simulink model "FOCControlDiscreteModel"  (R2022a)
settings: Solver=FixedStepDiscrete  StartTime=0.0  StopTime=2  RelTol=1e-3  EnableMultiTasking=on
values from neighbouring files (symbols this model uses):
  Ki_current = 6.0    (= 6)    [FOCControlDiscrete.m]
  Ki_speed = 6.0    (= 6)    [FOCControlDiscrete.m]
  Kp_current = 12.0    (= 12)    [FOCControlDiscrete.m]
  Kp_speed = 0.459    [FOCControlDiscrete.m]
  P = 6    [FOCControlDiscrete.m]
  Ts_current_control_loop = 30e-6    (= 3e-05)    [FOCControlDiscrete.m]
  Ts_speed_control_loop = 2 * Ts_observer    (= 0.00012)    [FOCControlDiscrete.m]
  Vdc = 12    [FOCControlDiscrete.m]
undefined symbols (not defined in the file or in its folder): Ts_motor
libraries: mcbcontrolslib x6, slpidlib x3, mcbpositiondecoderlib x3, simulink_extras x2, mcbplantlib x1, autolibpmsmexterior x1
settings Model: Creator=brandon  LastModifiedBy=brandon
settings SolverCC: AutoInsertRateTranBlk=on
settings DebuggingCC: ParameterPrecisionLossMsg=none

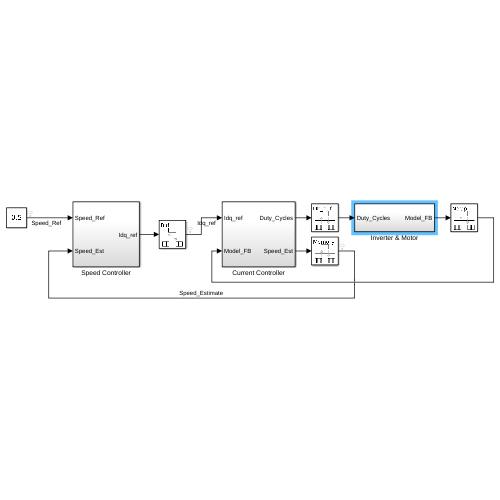
[thumbnail: Simulink's stored preview of the top-level diagram]
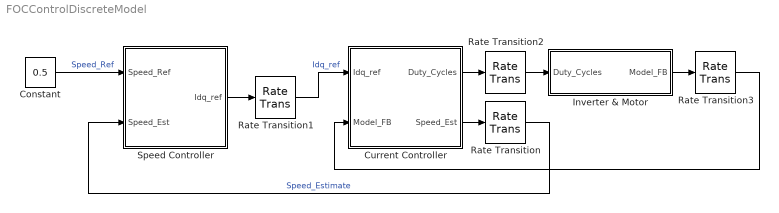
== system FOCControlDiscreteModel ==
  Constant : Constant  Value=0.5  OutDataTypeStr=single
  Current Controller : Subsystem
  Inverter & Motor : Subsystem
  Rate Transition{,1..3} (4 alike) : RateTransition  Deterministic=off
  Speed Controller : Subsystem
  wires:
  Constant/1 -> Speed Controller/1(Speed_Ref)  "Speed_Ref"
  Rate Transition/1 -> Speed Controller/2(Speed_Est)  "Speed_Estimate"
  Speed Controller/1(Idq_ref) -> Rate Transition1/1
  Rate Transition1/1 -> Current Controller/1(Idq_ref)  "Idq_ref"
  Current Controller/1(Duty_Cycles) -> Rate Transition2/1
  Rate Transition2/1 -> Inverter & Motor/1(Duty_Cycles)
  Inverter & Motor/1(Model_FB) -> Rate Transition3/1
  Rate Transition3/1 -> Current Controller/2(Model_FB)
  Current Controller/2(Speed_Est) -> Rate Transition/1

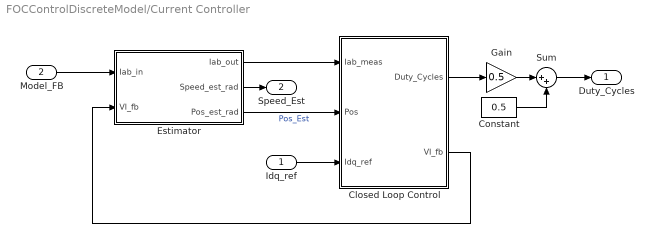
== system FOCControlDiscreteModel/Current Controller ==
  Idq_ref : Inport
  Model_FB : Inport  Port=2
  Closed Loop Control : Subsystem
  Constant : Constant  Value=0.5  OutDataTypeStr=single
  Estimator : Subsystem
  Gain : Gain  Gain=0.5  OutDataTypeStr=single
  Sum : Sum  Inputs=|++
  Duty_Cycles : Outport
  Speed_Est : Outport  Port=2
  wires:
  Model_FB/1 -> Estimator/1(Iab_in)
  Closed Loop Control/2(VI_fb) -> Estimator/2(VI_fb)
  Estimator/2(Speed_est_rad) -> Speed_Est/1
  Estimator/3(Pos_est_rad) -> Closed Loop Control/2(Pos)  "Pos_Est"
  Estimator/1(Iab_out) -> Closed Loop Control/1(Iab_meas)
  Idq_ref/1 -> Closed Loop Control/3(Idq_ref)
  Closed Loop Control/1(Duty_Cycles) -> Gain/1
  Gain/1 -> Sum/1
  Constant/1 -> Sum/2
  Sum/1 -> Duty_Cycles/1

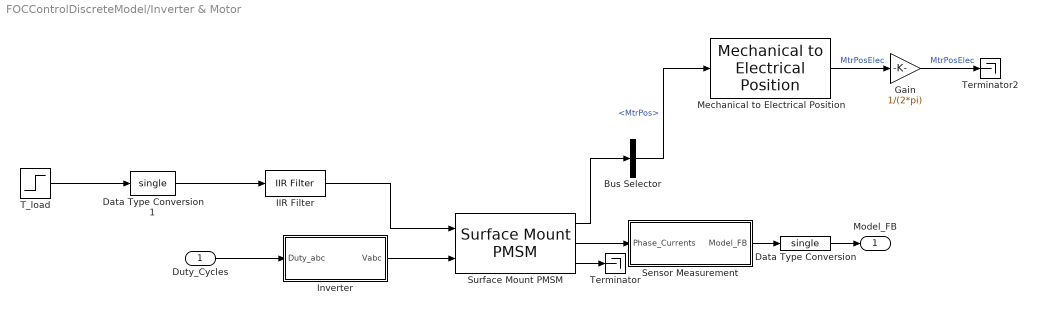
== system FOCControlDiscreteModel/Inverter & Motor ==
  Duty_Cycles : Inport
  Bus Selector : BusSelector  OutputSignals=MtrPos
  Data Type Conversion : DataTypeConversion  OutDataTypeStr=single  SaturateOnIntegerOverflow=off  RndMeth=Floor
  Data Type Conversion1 : DataTypeConversion  OutDataTypeStr=single  SaturateOnIntegerOverflow=off  RndMeth=Floor
  Gain : Gain  Gain=1/(2*pi)  OutDataTypeStr=Inherit: Same as input
  IIR Filter : mcbcontrolslib/IIR Filter  VariantControl=Low Pass Filter  VariantSelect=Low-pass  Filter_constant=0.0001  advancedSettings=on  Ts=50e-6  cutOff_freq=0.31834
      settings: SourceProductBaseCode=MT
  Inverter : Subsystem
  Mechanical to Electrical Position : mcbpositiondecoderlib/Mechanical to Electrical Position  NrPP=P  selectedRange=Radians  MechOfstInputType=Specify via dialog  mechOffsetIn=0  maxAngleIn=2*pi  InputDataType=single  VariantSelect=floating-point
      settings: SourceProductBaseCode=MT
  Sensor Measurement : Subsystem
  Surface Mount PMSM : autolibpmsmexterior/Surface Mount PMSM  port_config=Torque  sim_type=Discrete  Ts=Ts_motor  P=P  Rs=Rs  Ldq_=Ls  KConstText=Permanent flux linkage constant (lambda_pm):  lambda_pm=Psi  Ke=159.9771  Kt=1.323  mechanical=[0.0027, 4.924e-4, 0]  idq0=[0 0]  theta_init=0  omega_init=0  KConst=Psi  lambda_pm_calc=Psi  RefBlkName='autolibpmsmexterior/Surface Mount PMSM'  aMode=5  Ldq="[0.0017      0.0017]"
      settings: SourceProductBaseCode=PW,DR,MT,VE
  T_load : Step  Time=4  Before=0.0001  After=0.005  SampleTime=Ts_speed_control_loop
  Terminator : Terminator
  Terminator2 : Terminator
  Model_FB : Outport
  wires:
  Duty_Cycles/1 -> Inverter/1(Duty_abc)
  IIR Filter/1 -> Surface Mount PMSM/1
  Inverter/1(Vabc) -> Surface Mount PMSM/2
  Surface Mount PMSM/3 -> Terminator/1
  Surface Mount PMSM/1 -> Bus Selector/1
  Surface Mount PMSM/2 -> Sensor Measurement/1(Phase_Currents)
  Sensor Measurement/1(Model_FB) -> Data Type Conversion/1
  Data Type Conversion/1 -> Model_FB/1
  T_load/1 -> Data Type Conversion1/1
  Data Type Conversion1/1 -> IIR Filter/1
  Mechanical to Electrical Position/1 -> Gain/1  "MtrPosElec"
  Gain/1 -> Terminator2/1  "MtrPosElec"
  Bus Selector/1 -> Mechanical to Electrical Position/1  "<MtrPos>"

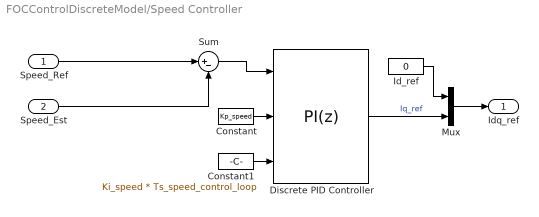
== system FOCControlDiscreteModel/Speed Controller ==
  Speed_Ref : Inport
  Speed_Est : Inport  Port=2
  Constant : Constant  Value=Kp_speed  OutDataTypeStr=single
  Constant1 : Constant  Value=Ki_speed * Ts_speed_control_loop  OutDataTypeStr=single
  Discrete PID Controller : slpidlib/PID Controller  Controller=PI  Form=Parallel  TimeDomain=Discrete-time  UseExternalTs=off  SampleTime=-1  IntegratorMethod=Forward Euler  FilterMethod=Forward Euler  ControllerParametersSource=external  P=1  I=1  UseKiTs=on  D=0  N=100  UseFilter=off  TunerSelectOption=Transfer Function Based (PID Tuner App)  ZeroCross=off  InitialConditionSource=internal  InitialConditionForIntegrator=0  InitialConditionForFilter=0  DifferentiatorICPrevScaledInput=0  ExternalReset=none  TrackingMode=off  Kt=1  LimitOutput=on  SatLimitsSource=internal  UpperSaturationLimit=10  LowerSaturationLimit=-10  LinearizeAsGain=off  AntiWindupMode=clamping  Kb=1  PGainOutDataTypeStr=single  PProdOutDataTypeStr=single  POutMin=[]  POutMax=[]  IGainOutDataTypeStr=single  IProdOutDataTypeStr=single  IOutMin=[]  IOutMax=[]  DGainOutDataTypeStr=single  DProdOutDataTypeStr=single  DOutMin=[]  DOutMax=[]  NOutMin=[]  NOutMax=[]  SumOutDataTypeStr=single  SumOutMin=[]  SumOutMax=[]  SaturationOutDataTypeStr=single  SaturationOutMin=[]  SaturationOutMax=[]  PParamMin=[]  PParamMax=[]  IParamMin=[]  IParamMax=[]  DParamMin=[]  DParamMax=[]  NParamMin=[]  NParamMax=[]  KbParamMin=[]  KbParamMax=[]  KtParamMin=[]  KtParamMax=[]  KbOutMin=[]  KbOutMax=[]  KtOutMin=[]  KtOutMax=[]  IntegratorOutDataTypeStr=single  IntegratorOutMin=[]  IntegratorOutMax=[]  FilterOutMin=[]  FilterOutMax=[]  SumI1OutMin=[]  SumI1OutMax=[]  SumI2OutMin=[]  SumI2OutMax=[]  SumI3OutMin=[]  SumI3OutMax=[]  SumI4OutMin=[]  SumI4OutMax=[]  SumDOutMin=[]  SumDOutMax=[]  SumAccumDataTypeStr=single  DifferentiatorOutDataTypeStr=single  DifferentiatorOutMin=[]  DifferentiatorOutMax=[]  FilterDiffOutCoefMin=[]  FilterDiffOutCoefMax=[]  ReciprocalOutMin=[]  ReciprocalOutMax=[]  SumDenOutMin=[]  SumDenOutMax=[]  SumNumOutMin=[]  SumNumOutMax=[]  DivideOutMin=[]  DivideOutMax=[]  UdiffTsProdOutMin=[]  UdiffTsProdOutMax=[]  NTsProdOutMin=[]  NTsProdOutMax=[]  UintegralTsProdOutMin=[]  UintegralTsProdOutMax=[]  UngainTsProdOutMin=[]  UngainTsProdOutMax=[]  IntegratorContinuousStateAttributes=''  IntegratorStateMustResolveToSignalObject=off  IntegratorRTWStateStorageClass=Auto  FilterContinuousStateAttributes=''  FilterStateMustResolveToSignalObject=off  FilterRTWStateStorageClass=Auto  ParallelPVariant=ExternalParameters  IdealPVariant=Disabled  IVariant=ExternalParameters  DVariant=Disabled  IntegratorVariant=Discrete  SatVariant=Enabled  AWVariant=DiscClampingParallel  PCopyVariant=Disabled  TRVariant=Disabled  FdbkBlocksVariant=Forward  IdealPFdbkVariant=Disabled  SatFdbkVariant=Disabled  DerivativeFilterVariant=Disabled  NVariant=Disabled  NCopyVariant=Disabled_SignalSpec  FilterICVariant=Disabled  IntegratorICVariant=InternalICs  ExternalResetVariant=Disabled  TRSumVariant=Passthrough  SumFdbkVariant=Disabled  SumVariant=Sum_PI  TsampFilterVariant=InternalTs  TsampNgainVariant=Passthrough  TsampIntegralVariant=Passthrough  ExternalSaturationOutDataTypeStr=Inherit: Same as second input  aMode=0
  Id_ref : Constant  Value=0  OutDataTypeStr=single
  Mux : Mux  Inputs=2
  Sum : Sum  Inputs=|+-
  Idq_ref : Outport
  wires:
  Speed_Est/1 -> Sum/2
  Speed_Ref/1 -> Sum/1
  Discrete PID Controller/1 -> Mux/2  "Iq_ref"
  Sum/1 -> Discrete PID Controller/1
  Constant/1 -> Discrete PID Controller/2
  Constant1/1 -> Discrete PID Controller/3
  Id_ref/1 -> Mux/1
  Mux/1 -> Idq_ref/1

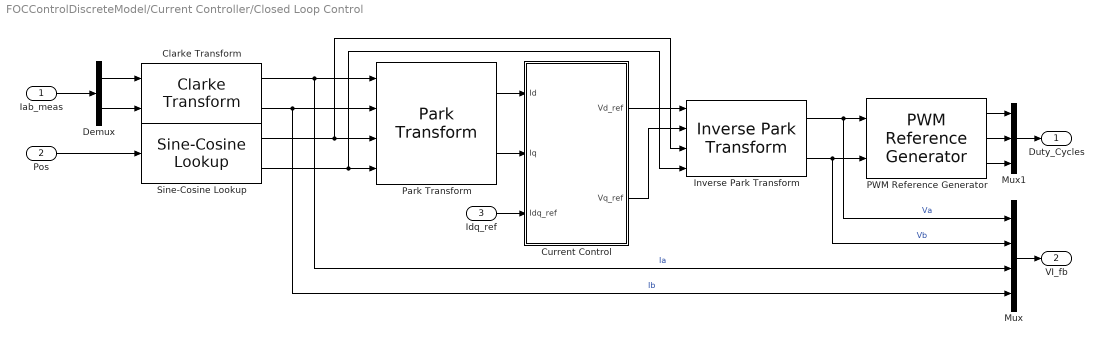
== system FOCControlDiscreteModel/Current Controller/Closed Loop Control ==
  Iab_meas : Inport
  Pos : Inport  Port=2
  Idq_ref : Inport  Port=3
  Clarke Transform : mcbcontrolslib/Clarke Transform  VariantControl=Variant2
  Current Control : Subsystem
  Demux : Demux  Outputs=2
  Inverse Park Transform : mcbcontrolslib/Inverse Park Transform  AxisAlignment=D-axis
  Mux : Mux
  Mux1 : Mux  Inputs=3
  PWM Reference Generator : mcbcontrolslib/PWM Reference Generator  inSignal=Valphabeta  modType=SVM: space vector modulation
      settings: SourceProductBaseCode=MT
  Park Transform : mcbcontrolslib/Park Transform  AxisAlignment=D-axis
      settings: SourceProductBaseCode=MT
  Sine-Cosine Lookup : mcbcontrolslib/Sine-Cosine Lookup  AngleInput=Radians  N_points=1024
      settings: SourceProductBaseCode=MT
  Duty_Cycles : Outport
  VI_fb : Outport  Port=2
  wires:
  Pos/1 -> Sine-Cosine Lookup/1
  Iab_meas/1 -> Demux/1
  Demux/1 -> Clarke Transform/1
  Demux/2 -> Clarke Transform/2
  Clarke Transform/2 -> Mux/4, Park Transform/2  "Ib"
  Clarke Transform/1 -> Mux/3, Park Transform/1  "Ia"
  Sine-Cosine Lookup/1 -> Park Transform/3, Inverse Park Transform/3
  Sine-Cosine Lookup/2 -> Park Transform/4, Inverse Park Transform/4
  Park Transform/1 -> Current Control/1(Id)
  Park Transform/2 -> Current Control/2(Iq)
  Idq_ref/1 -> Current Control/3(Idq_ref)
  Current Control/1(Vd_ref) -> Inverse Park Transform/1
  Current Control/2(Vq_ref) -> Inverse Park Transform/2
  Inverse Park Transform/2 -> Mux/2, PWM Reference Generator/2  "Vb"
  Inverse Park Transform/1 -> Mux/1, PWM Reference Generator/1  "Va"
  PWM Reference Generator/1 -> Mux1/1
  PWM Reference Generator/2 -> Mux1/2
  PWM Reference Generator/3 -> Mux1/3
  Mux1/1 -> Duty_Cycles/1
  Mux/1 -> VI_fb/1

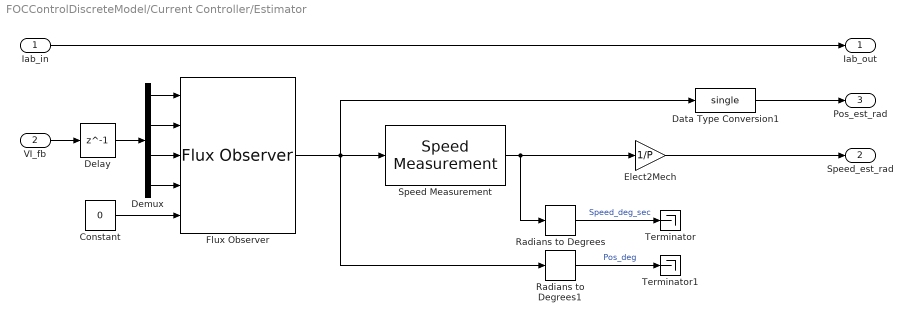
== system FOCControlDiscreteModel/Current Controller/Estimator ==
  Iab_in : Inport
  VI_fb : Inport  Port=2
  Constant : Constant  Value=0  OutDataTypeStr=single
  Data Type Conversion1 : DataTypeConversion  OutDataTypeStr=single  SaturateOnIntegerOverflow=off  RndMeth=Floor
  Delay : Delay  DelayLength=1  InitialCondition=0
  Demux : Demux
  Elect2Mech : Gain  Gain=1/P
  Flux Observer : mcbpositiondecoderlib/Flux Observer  MotorSelection=PMSM  BlockInputUnit=SI unit  PerUnitVoltage=13.86  PerUnitCurrent=19.3  PositionSelect=on  FluxSelect=off  TorqueSelect=off  PolePairs=4  StatorResistance=Rs  StatorDAxisInductance=Ls  StatorLeakageInductance=0.0068  RotorLeakageInductance=0.0068  MagnetizingInductance=0.0300  CutoffFreq=1  BlockSampleTime=Ts_observer  PositionUnit=Radians  PositionDatatype=double  FluxUnit=Weber  PerUnitFlux=0.1  FluxDatatype=single  TorqueUnit=Nm  PerUnitTorque=100  TorqueDatatype=single
      settings: SourceProductBaseCode=MT
  Radians to Degrees : simulink_extras/Transformations/Radians to Degrees
  Radians to Degrees1 : simulink_extras/Transformations/Radians to Degrees
  Speed Measurement : mcbpositiondecoderlib/Speed Measurement  PositionUnit=Radians  PositionScalingDatatype=uint32  SpeedCalculationMode=Time interval for speed calculation  SampleTimeAsync=Ts_observer  MaximumApplicationSpeed=W_max_rpm  SpeedResolution=5e-6  DelayLength=10  MaximumMeasurableSpeed=49999  MeasurableSpeedResolution=2.3283e-05  SpeedUnit=Radians/Sec  PerUnitSpeed=1000  SpeedDataType=single
      settings: SourceProductBaseCode=MT
  Terminator : Terminator
  Terminator1 : Terminator
  Iab_out : Outport
  Speed_est_rad : Outport  Port=2
  Pos_est_rad : Outport  Port=3
  wires:
  Iab_in/1 -> Iab_out/1
  VI_fb/1 -> Delay/1
  Demux/4 -> Flux Observer/4
  Demux/3 -> Flux Observer/3
  Demux/2 -> Flux Observer/2
  Demux/1 -> Flux Observer/1
  Constant/1 -> Flux Observer/5
  Flux Observer/1 -> Radians to Degrees1/1, Data Type Conversion1/1, Speed Measurement/1
  Speed Measurement/1 -> Elect2Mech/1, Radians to Degrees/1
  Data Type Conversion1/1 -> Pos_est_rad/1
  Radians to Degrees/1 -> Terminator/1  "Speed_deg_sec"
  Radians to Degrees1/1 -> Terminator1/1  "Pos_deg"
  Elect2Mech/1 -> Speed_est_rad/1
  Delay/1 -> Demux/1

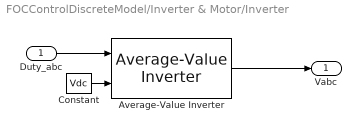
== system FOCControlDiscreteModel/Inverter & Motor/Inverter ==
  Duty_abc : Inport
  Average-Value Inverter : mcbplantlib/Average-Value Inverter
  Constant : Constant  Value=Vdc
  Vabc : Outport
  wires:
  Duty_abc/1 -> Average-Value Inverter/1
  Average-Value Inverter/1 -> Vabc/1
  Constant/1 -> Average-Value Inverter/2

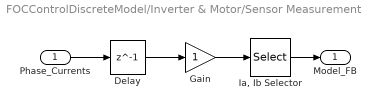
== system FOCControlDiscreteModel/Inverter & Motor/Sensor Measurement ==
  Phase_Currents : Inport
  Delay : Delay  DelayLength=1  InitialCondition=0
  Gain : Gain
  "Ia, Ib Selector" : Selector  InputPortWidth=3  IndexOptions=Index vector (dialog)  Indices=[1 2]  OutputSizes=1
  Model_FB : Outport
  wires:
  Phase_Currents/1 -> Delay/1
  Delay/1 -> Gain/1
  Gain/1 -> "Ia, Ib Selector"/1
  "Ia, Ib Selector"/1 -> Model_FB/1

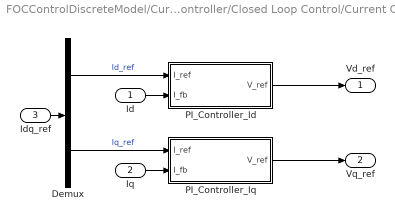
== system FOCControlDiscreteModel/Current Controller/Closed Loop Control/Current Control ==
  Id : Inport
  Iq : Inport  Port=2
  Idq_ref : Inport  Port=3
  Demux : Demux  Outputs=2
  PI_Controller_Id : Subsystem
  PI_Controller_Iq : Subsystem
  Vd_ref : Outport
  Vq_ref : Outport  Port=2
  wires:
  PI_Controller_Iq/1(V_ref) -> Vq_ref/1
  PI_Controller_Id/1(V_ref) -> Vd_ref/1
  Id/1 -> PI_Controller_Id/2(I_fb)
  Iq/1 -> PI_Controller_Iq/2(I_fb)
  Demux/1 -> PI_Controller_Id/1(I_ref)  "Id_ref"
  Demux/2 -> PI_Controller_Iq/1(I_ref)  "Iq_ref"
  Idq_ref/1 -> Demux/1

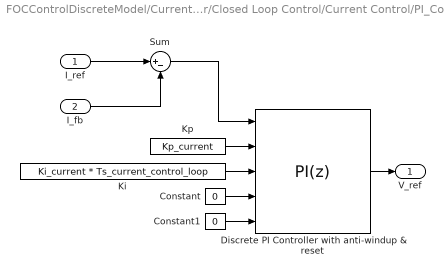
== system FOCControlDiscreteModel/Current Controller/Closed Loop Control/Current Control/PI_Controller_Id ==
  I_ref : Inport
  I_fb : Inport  Port=2
  Constant : Constant  Value=0  OutDataTypeStr=single
  Constant1 : Constant  Value=0  OutDataTypeStr=single
  Discrete PI Controller with anti-windup & reset : slpidlib/PID Controller  Controller=PI  Form=Parallel  TimeDomain=Discrete-time  UseExternalTs=off  SampleTime=-1  IntegratorMethod=Forward Euler  FilterMethod=Forward Euler  ControllerParametersSource=external  P=1  I=1  UseKiTs=on  D=0  N=100  UseFilter=on  TunerSelectOption=Transfer Function Based (PID Tuner App)  InitialConditionSource=external  InitialConditionForIntegrator=0  InitialConditionForFilter=0  DifferentiatorICPrevScaledInput=0  ExternalReset=level  TrackingMode=off  Kt=1  LimitOutput=on  SatLimitsSource=internal  UpperSaturationLimit=1  LowerSaturationLimit=-1  LinearizeAsGain=on  AntiWindupMode=clamping  Kb=1  RndMeth=Simplest  POutMin=[]  POutMax=[]  IOutMin=[]  IOutMax=[]  DOutMin=[]  DOutMax=[]  NOutMin=[]  NOutMax=[]  SumOutMin=[]  SumOutMax=[]  SaturationOutDataTypeStr=Inherit: Inherit via back propagation  SaturationOutMin=[]  SaturationOutMax=[]  PParamMin=[]  PParamMax=[]  IParamMin=[]  IParamMax=[]  DParamMin=[]  DParamMax=[]  NParamMin=[]  NParamMax=[]  KbParamMin=[]  KbParamMax=[]  KtParamMin=[]  KtParamMax=[]  KbOutMin=[]  KbOutMax=[]  KtOutMin=[]  KtOutMax=[]  IntegratorOutMin=[]  IntegratorOutMax=[]  FilterOutMin=[]  FilterOutMax=[]  SumI1OutMin=[]  SumI1OutMax=[]  SumI2OutMin=[]  SumI2OutMax=[]  SumI3OutMin=[]  SumI3OutMax=[]  SumI4OutMin=[]  SumI4OutMax=[]  SumDOutMin=[]  SumDOutMax=[]  DifferentiatorOutMin=[]  DifferentiatorOutMax=[]  FilterDiffOutCoefMin=[]  FilterDiffOutCoefMax=[]  ReciprocalOutMin=[]  ReciprocalOutMax=[]  SumDenOutMin=[]  SumDenOutMax=[]  SumNumOutMin=[]  SumNumOutMax=[]  DivideOutMin=[]  DivideOutMax=[]  UdiffTsProdOutMin=[]  UdiffTsProdOutMax=[]  NTsProdOutMin=[]  NTsProdOutMax=[]  UintegralTsProdOutMin=[]  UintegralTsProdOutMax=[]  UngainTsProdOutMin=[]  UngainTsProdOutMax=[]  IntegratorContinuousStateAttributes=''  IntegratorStateMustResolveToSignalObject=off  IntegratorRTWStateStorageClass=Auto  FilterContinuousStateAttributes=''  FilterStateMustResolveToSignalObject=off  FilterRTWStateStorageClass=Auto  ParallelPVariant=ExternalParameters  IdealPVariant=Disabled  IVariant=ExternalParameters  DVariant=Disabled  IntegratorVariant=Discrete  SatVariant=Enabled  AWVariant=DiscClampingParallel  PCopyVariant=Disabled  TRVariant=Disabled  FdbkBlocksVariant=Forward  IdealPFdbkVariant=Disabled  SatFdbkVariant=Disabled  DerivativeFilterVariant=Disabled  NVariant=Disabled  NCopyVariant=Disabled_SignalSpec  FilterICVariant=Disabled  IntegratorICVariant=ExternalICs  ExternalResetVariant=ExternalReset  TRSumVariant=Passthrough  SumFdbkVariant=Disabled  SumVariant=Sum_PI  TsampFilterVariant=InternalTs  TsampNgainVariant=Passthrough  TsampIntegralVariant=Passthrough  ExternalSaturationOutDataTypeStr=Inherit: Same as second input  aMode=5
  Ki : Constant  Value=Ki_current * Ts_current_control_loop  OutDataTypeStr=single  SampleTime=-1
  Kp : Constant  Value=Kp_current  OutDataTypeStr=single  SampleTime=-1
  Sum : Sum  Inputs=|+-  OutDataTypeStr=Inherit: Same as first input
  V_ref : Outport
  wires:
  Ki/1 -> Discrete PI Controller with anti-windup & reset/3
  I_ref/1 -> Sum/1
  Kp/1 -> Discrete PI Controller with anti-windup & reset/2
  Sum/1 -> Discrete PI Controller with anti-windup & reset/1
  I_fb/1 -> Sum/2
  Discrete PI Controller with anti-windup & reset/1 -> V_ref/1
  Constant1/1 -> Discrete PI Controller with anti-windup & reset/5
  Constant/1 -> Discrete PI Controller with anti-windup & reset/4

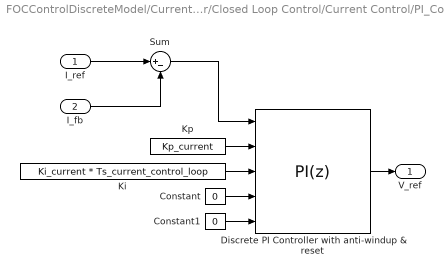
== system FOCControlDiscreteModel/Current Controller/Closed Loop Control/Current Control/PI_Controller_Iq ==
  I_ref : Inport
  I_fb : Inport  Port=2
  Constant : Constant  Value=0  OutDataTypeStr=single
  Constant1 : Constant  Value=0  OutDataTypeStr=single
  Discrete PI Controller with anti-windup & reset : slpidlib/PID Controller  Controller=PI  Form=Parallel  TimeDomain=Discrete-time  UseExternalTs=off  SampleTime=-1  IntegratorMethod=Forward Euler  FilterMethod=Forward Euler  ControllerParametersSource=external  P=1  I=1  UseKiTs=on  D=0  N=100  UseFilter=on  TunerSelectOption=Transfer Function Based (PID Tuner App)  InitialConditionSource=external  InitialConditionForIntegrator=0  InitialConditionForFilter=0  DifferentiatorICPrevScaledInput=0  ExternalReset=level  TrackingMode=off  Kt=1  LimitOutput=on  SatLimitsSource=internal  UpperSaturationLimit=1  LowerSaturationLimit=-1  LinearizeAsGain=on  AntiWindupMode=clamping  Kb=1  RndMeth=Simplest  POutMin=[]  POutMax=[]  IOutMin=[]  IOutMax=[]  DOutMin=[]  DOutMax=[]  NOutMin=[]  NOutMax=[]  SumOutMin=[]  SumOutMax=[]  SaturationOutDataTypeStr=Inherit: Inherit via back propagation  SaturationOutMin=[]  SaturationOutMax=[]  PParamMin=[]  PParamMax=[]  IParamMin=[]  IParamMax=[]  DParamMin=[]  DParamMax=[]  NParamMin=[]  NParamMax=[]  KbParamMin=[]  KbParamMax=[]  KtParamMin=[]  KtParamMax=[]  KbOutMin=[]  KbOutMax=[]  KtOutMin=[]  KtOutMax=[]  IntegratorOutMin=[]  IntegratorOutMax=[]  FilterOutMin=[]  FilterOutMax=[]  SumI1OutMin=[]  SumI1OutMax=[]  SumI2OutMin=[]  SumI2OutMax=[]  SumI3OutMin=[]  SumI3OutMax=[]  SumI4OutMin=[]  SumI4OutMax=[]  SumDOutMin=[]  SumDOutMax=[]  DifferentiatorOutMin=[]  DifferentiatorOutMax=[]  FilterDiffOutCoefMin=[]  FilterDiffOutCoefMax=[]  ReciprocalOutMin=[]  ReciprocalOutMax=[]  SumDenOutMin=[]  SumDenOutMax=[]  SumNumOutMin=[]  SumNumOutMax=[]  DivideOutMin=[]  DivideOutMax=[]  UdiffTsProdOutMin=[]  UdiffTsProdOutMax=[]  NTsProdOutMin=[]  NTsProdOutMax=[]  UintegralTsProdOutMin=[]  UintegralTsProdOutMax=[]  UngainTsProdOutMin=[]  UngainTsProdOutMax=[]  IntegratorContinuousStateAttributes=''  IntegratorStateMustResolveToSignalObject=off  IntegratorRTWStateStorageClass=Auto  FilterContinuousStateAttributes=''  FilterStateMustResolveToSignalObject=off  FilterRTWStateStorageClass=Auto  ParallelPVariant=ExternalParameters  IdealPVariant=Disabled  IVariant=ExternalParameters  DVariant=Disabled  IntegratorVariant=Discrete  SatVariant=Enabled  AWVariant=DiscClampingParallel  PCopyVariant=Disabled  TRVariant=Disabled  FdbkBlocksVariant=Forward  IdealPFdbkVariant=Disabled  SatFdbkVariant=Disabled  DerivativeFilterVariant=Disabled  NVariant=Disabled  NCopyVariant=Disabled_SignalSpec  FilterICVariant=Disabled  IntegratorICVariant=ExternalICs  ExternalResetVariant=ExternalReset  TRSumVariant=Passthrough  SumFdbkVariant=Disabled  SumVariant=Sum_PI  TsampFilterVariant=InternalTs  TsampNgainVariant=Passthrough  TsampIntegralVariant=Passthrough  ExternalSaturationOutDataTypeStr=Inherit: Same as second input  aMode=5
  Ki : Constant  Value=Ki_current * Ts_current_control_loop  OutDataTypeStr=single  SampleTime=-1
  Kp : Constant  Value=Kp_current  OutDataTypeStr=single  SampleTime=-1
  Sum : Sum  Inputs=|+-  OutDataTypeStr=Inherit: Same as first input
  V_ref : Outport
  wires:
  Ki/1 -> Discrete PI Controller with anti-windup & reset/3
  I_ref/1 -> Sum/1
  Kp/1 -> Discrete PI Controller with anti-windup & reset/2
  Sum/1 -> Discrete PI Controller with anti-windup & reset/1
  I_fb/1 -> Sum/2
  Discrete PI Controller with anti-windup & reset/1 -> V_ref/1
  Constant1/1 -> Discrete PI Controller with anti-windup & reset/5
  Constant/1 -> Discrete PI Controller with anti-windup & reset/4
